simulink model "single_engine_LQG_250120"  (R2018b)
settings: Solver=VariableStepAuto  StartTime=0.0  StopTime=10.0  FixedStep=0.001  RelTol=1e-3
values from neighbouring files (symbols this model uses):
  A = J*(Omega_phi + Omega)    [IMU.m]
  D = simplify(D)    [dynamika_gimbala_symbolicznie.m]    (also in dynamika_gimbala_symbolicznie_20190706.m; dynamika_gimbala_symbolicznie_20190825.m; gimbal_dynamics.m = calculate_D_matrix(THETA,I1,I2,I3,DIM))
undefined symbols (not defined in the file or in its folder): B, C, Continuous, Time
libraries: ctrlSharedLib x1
settings Model: Creator=Paweł Tymiński  LastModifiedBy=Paweł Tymiński

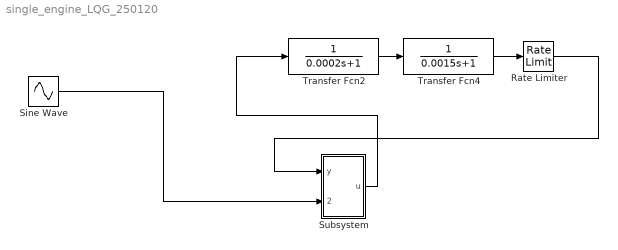
== system single_engine_LQG_250120 ==
  Rate Limiter : RateLimiter  RisingSlewLimit=18.5  FallingSlewLimit=-18.5  SampleTimeMode=inherited
  Sine Wave : Sin  Frequency=10  SampleTime=0
  Subsystem : Subsystem
  Transfer Fcn2 : TransferFcn  Denominator=[0.0002 1]
  Transfer Fcn4 : TransferFcn  Denominator=[0.0015 1]
  wires:
  Transfer Fcn4/1 -> Rate Limiter/1
  Transfer Fcn2/1 -> Transfer Fcn4/1
  Rate Limiter/1 -> Subsystem/1(y)
  Sine Wave/1 -> Subsystem/2(y_zad)
  Subsystem/1(u) -> Transfer Fcn2/1

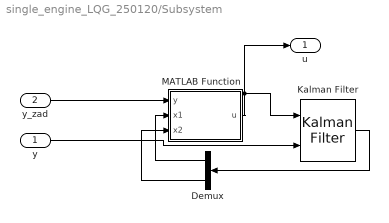
== system single_engine_LQG_250120/Subsystem ==
  y : Inport
  y_zad : Inport  Port=2
  Demux : Demux  Outputs=2
  Kalman Filter : ctrlSharedLib/Kalman Filter  TimeDomain=Continuous-Time  UseCurrentEstimator=on  ModelSource=Individual A, B, C, D matrices  ModelSourceVariable=ss(0.95,1,1,0,1)  A=A  B=B  C=C  D=D  NumberOfStates=1  NumberOfInputs=1  NumberOfOutputs=1  InitialEstimateSource=Dialog  X0=0  P0=10  UseK=off  UseGH=off  NumberOfProcessNoiseInputs=1  G=1  TimeInvariantG=on  H=0  TimeInvariantH=on  Q=30000  TimeInvariantQ=on  R=0.01  TimeInvariantR=on  N=0  TimeInvariantN=on  AddInputPort=on  AddEnablePort=off  OutputEstimatedY=off  OutputP=off  Ts=0.001
      settings: SourceProductBaseCode=CT
  MATLAB Function : MATLAB Function  TreatAsAtomicUnit=on
  u : Outport
  wires:
  MATLAB Function/1(u) -> u/1, Kalman Filter/1
  Kalman Filter/1 -> Demux/1
  Demux/1 -> MATLAB Function/2(x1)
  Demux/2 -> MATLAB Function/3(x2)
  y/1 -> Kalman Filter/2
  y_zad/1 -> MATLAB Function/1(y)

== matlab function single_engine_LQG_250120/Subsystem/MATLAB Function ==
  data: y input; u output; x1 input; x2 input
function u = fcn(y,x1,x2)
K =[0.0045    0.0102];
Nu=1;
Nx =[0; 0.0492];
u=-K*[x1;x2]+(Nu+K*Nx)*y;
